simulink library "csu_tdl_thruster_dynamics_lander_lib"  (R2014b)
settings: Solver=ode45  StartTime=0.0  StopTime=10.0  RelTol=1e-3
values from neighbouring files (symbols this model uses):
  sim_time_step_size = 0.01    [csu_tdl_thruster_dynamics_lander_test.m]    (also in sim_thruster_wsim_test.m)
  tdl_active_time = 0.9/1000    (= 0.0009)    [csu_tdl_thruster_dynamics_lander_init.m]
undefined symbols (not defined in the file or in its folder): tdl_valve_delay_cycles
libraries: simulink x7, util_event_lib x2, util_info_lib x1, util_common_lib x1
settings Model: Creator=Nilesh  LastModifiedBy=mstewart

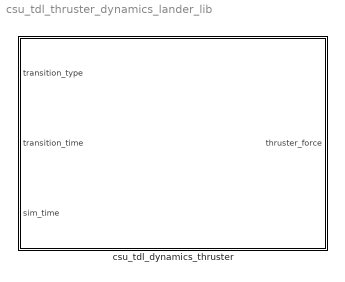
== system csu_tdl_thruster_dynamics_lander_lib ==
  csu_tdl_dynamics_thruster : Subsystem  mask{thruster_idx=[], num_thrusters=[], time_since_rise_lookup=[], thrust_rising_output_lookup=[], time_since_fall_lookup=[], thrust_falling_output_lookup=[], thrust_noise_mean=[], thrust_noise_std=[], thrust_noise_seed=[], thrust_noise_on=[]}
      mask prompts: thruster_idx "Thruster Index (1-total)"; num_thrusters "Number of thrusters (total)"; time_since_rise_lookup "Rising Transition: time vector for lookup table (seconds)"; thrust_rising_output_lookup "Rising Transition: thrust vector for lookup table (Newtons)"; time_since_fall_lookup "Falling Transition: time vector for lookup table (seconds)"; thrust_falling_output_lookup "Falling Transition: thrust vector for lookup table (Newtons)"; thrust_noise_mean "Output noise: bias in Newtons"; thrust_noise_std "Output noise: standard deviation in Newtons"; thrust_noise_seed "Output noise: random seed"; thrust_noise_on "Outpur noise Enabled (1 is noisy, 0 is clean)"

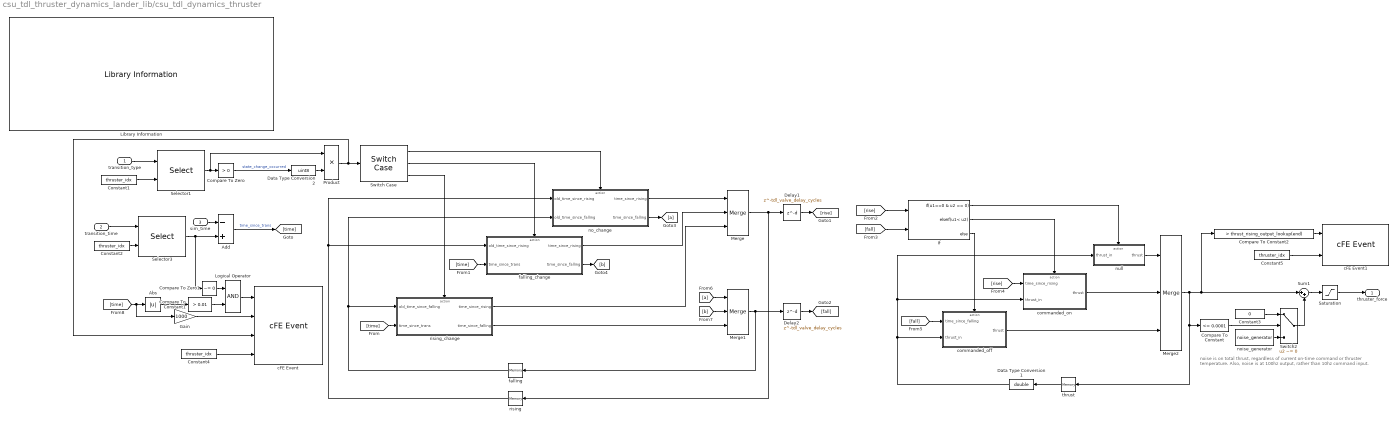
== system csu_tdl_thruster_dynamics_lander_lib/csu_tdl_dynamics_thruster ==
  note: noise is on total thrust, regardless of current on-time
      | command or thruster temperature. Also, noise is at 100hz output,
      | rather than 10hz command input.
  transition_type : Inport
  transition_time : Inport  Port=2
  sim_time : Inport  Port=3
  Abs : Abs
  Add : Sum  Inputs=-+
  Compare To Constant : simulink/Logic and Bit Operations/Compare To Constant  relop=<=  const=0.0001  OutDataTypeStr=boolean
  Compare To Constant1 : simulink/Logic and Bit Operations/Compare To Constant  relop=>  const=0.01  OutDataTypeStr=boolean
  Compare To Constant2 : simulink/Logic and Bit Operations/Compare To Constant  relop=>  const=thrust_rising_output_lookup(end)  OutDataTypeStr=boolean
  Compare To Zero : simulink/Logic and Bit Operations/Compare To Zero  relop=>  OutDataTypeStr=boolean
  Compare To Zero1 : simulink/Logic and Bit Operations/Compare To Zero  relop=~=  OutDataTypeStr=boolean
  Constant{1..2,4..5} (4 alike) : Constant  Value=thruster_idx  OutDataTypeStr=uint8
  Constant3 : Constant  Value=0
  Data Type Conversion1 : DataTypeConversion  OutDataTypeStr=double
  Data Type Conversion2 : DataTypeConversion  OutDataTypeStr=uint8
  Delay1 : Delay  DelayLength=tdl_valve_delay_cycles
  Delay2 : Delay  DelayLength=tdl_valve_delay_cycles
  Gain : Gain  Gain=1000
  If : If  NumInputs=2  IfExpression=u1==0 & u2 == 0  ElseIfExpressions=u1< u2
  Library Information : util_info_lib/Library Information  owner='escrane'
  Logical Operator : Logic  AllPortsSameDT=off  OutDataTypeStr=boolean
  Merge : Merge  Inputs=3
  Merge1 : Merge  Inputs=3
  Merge2 : Merge  Inputs=3
  Product : Product
  Saturation : Saturate  UpperLimit=1e10  LowerLimit=0
  Selector1 : Selector  InputPortWidth=num_thrusters  IndexOptions=Index vector (port)  Indices=[1 3]
  Selector3 : Selector  InputPortWidth=num_thrusters  IndexOptions=Index vector (port)  Indices=[1 3]
  Sum1 : Sum  Inputs=|++
  Switch Case : SwitchCase  CaseConditions={0,1,2}  ShowDefaultCase=off
  Switch2 : Switch  Criteria=u2 ~= 0
  cFE Event : util_event_lib/cFE Event  event_message='Incorrect transition time %f milliseconds detected on transition type %u in thruster %u'  event_id=thruster_idx+20  event_severity=DEBUG  event_use_enums=off  event_enum_types={}
  cFE Event1 : util_event_lib/cFE Event  event_message='Large thrust output in thruster %u'  event_id=thruster_idx+50  event_severity=DEBUG  event_use_enums=off  event_enum_types={}
  commanded_off : Subsystem  TreatAsAtomicUnit=on
  commanded_on : Subsystem  TreatAsAtomicUnit=on
  falling : Memory  InheritSampleTime=on
  falling_change : Subsystem  TreatAsAtomicUnit=on
  no_change : Subsystem  TreatAsAtomicUnit=on
  noise_generator : util_common_lib/noise_generator  std_dev=thrust_noise_std  bias=thrust_noise_mean  seed=thrust_noise_seed  on=thrust_noise_on  sample_time=sim_time_step_size
  null : Subsystem  TreatAsAtomicUnit=on
  rising : Memory  InheritSampleTime=on
  rising_change : Subsystem  TreatAsAtomicUnit=on
  thrust : Memory  InheritSampleTime=on
  thruster_force : Outport
  wires:
  If/1 -> null/Action
  thrust/1 -> Data Type Conversion1/1
  null/1(thrust) -> Merge2/1
  commanded_on/1(thrust) -> Merge2/2
  commanded_off/1(thrust) -> Merge2/3
  If/2 -> commanded_on/Action
  Delay2/1 -> [fall]
  Delay1/1 -> [rise]
  Merge1/1 -> falling/1, Delay2/1
  Merge/1 -> rising/1, Delay1/1
  [b] -> Merge1/2
  falling_change/2(time_since_falling) -> [b]
  [a] -> Merge1/1
  no_change/2(time_since_falling) -> [a]
  no_change/1(time_since_rising) -> Merge/1
  [fall] -> commanded_off/1(time_since_falling)
  [rise] -> commanded_on/1(time_since_rising)
  If/3 -> commanded_off/Action
  [rise] -> If/1
  [fall] -> If/2
  sim_time/1 -> Add/1
  Compare To Zero/1 -> Data Type Conversion2/1  "state_change_occurred"
  Data Type Conversion2/1 -> Product/2
  Add/1 -> [time]  "time_since_trans"
  Product/1 -> cFE Event/3, Switch Case/1
  Switch Case/1 -> no_change/Action
  Switch Case/2 -> falling_change/Action
  Switch Case/3 -> rising_change/Action
  [time] -> rising_change/2(time_since_trans)
  [time] -> falling_change/2(time_since_trans)
  falling/1 -> rising_change/1(old_time_since_falling), no_change/2(old_time_since_falling)
  rising/1 -> falling_change/1(old_time_since_rising), no_change/1(old_time_since_rising)
  falling_change/1(time_since_rising) -> Merge/2
  rising_change/1(time_since_rising) -> Merge/3
  rising_change/2(time_since_falling) -> Merge1/3
  Constant2/1 -> Selector3/2
  transition_time/1 -> Selector3/1
  Selector3/1 -> Compare To Zero1/1, Add/2
  Constant1/1 -> Selector1/2
  transition_type/1 -> Selector1/1
  Selector1/1 -> Product/1, Compare To Zero/1
  Data Type Conversion1/1 -> commanded_off/2(thrust_in), commanded_on/2(thrust_in), null/1(thrust_in)
  Compare To Constant/1 -> Switch2/2
  noise_generator/1 -> Switch2/3
  Constant3/1 -> Switch2/1
  Sum1/1 -> Saturation/1
  Switch2/1 -> Sum1/2
  Saturation/1 -> thruster_force/1
  [time] -> Abs/1, Gain/1
  Abs/1 -> Compare To Constant1/1
  Compare To Zero1/1 -> Logical Operator/1
  Compare To Constant1/1 -> Logical Operator/2
  Logical Operator/1 -> cFE Event/1
  Constant4/1 -> cFE Event/4
  Merge2/1 -> Compare To Constant2/1, Sum1/1, thrust/1, Compare To Constant/1
  Compare To Constant2/1 -> cFE Event1/1
  Constant5/1 -> cFE Event1/2
  Gain/1 -> cFE Event/2

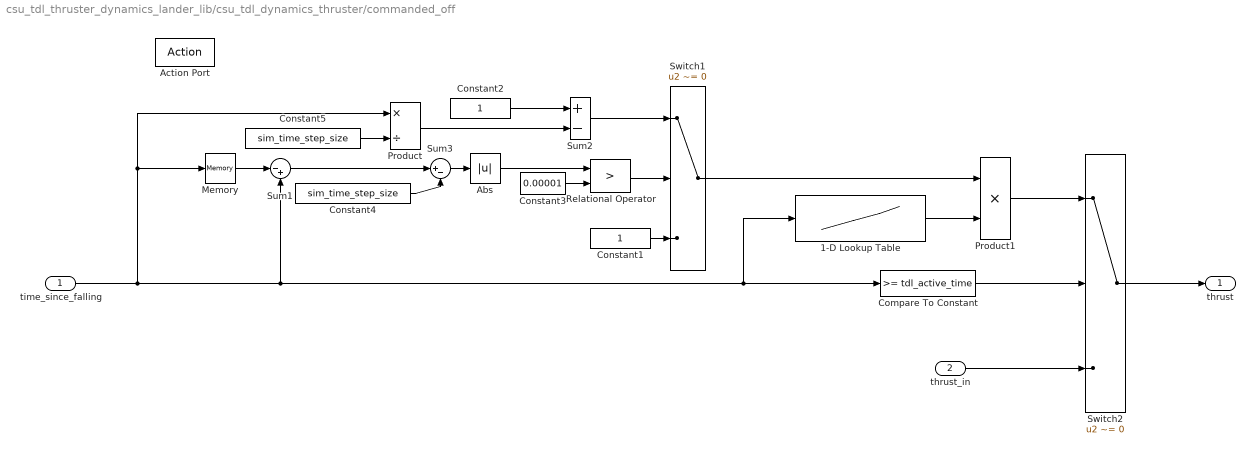
== system csu_tdl_thruster_dynamics_lander_lib/csu_tdl_dynamics_thruster/commanded_off ==
  time_since_falling : Inport
  thrust_in : Inport  Port=2
  Action Port : ActionPort
  1-D Lookup Table : Lookup_n-D  NumberOfTableDimensions=1  BreakpointsForDimension1=time_since_fall_lookup  BeginIndexSearchUsingPreviousIndexResult=on  Table=thrust_falling_output_lookup  ExtrapMethod=Clip  UseLastTableValue=on  InternalRulePriority=Speed  RndMeth=Simplest  InputSameDT=on
  Abs : Abs
  Compare To Constant : simulink/Logic and Bit Operations/Compare To Constant  relop=>=  const=tdl_active_time  OutDataTypeStr=boolean
  Constant1 : Constant
  Constant2 : Constant
  Constant3 : Constant  Value=0.00001  OutDataTypeStr=double
  Constant4 : Constant  Value=sim_time_step_size
  Constant5 : Constant  Value=sim_time_step_size
  Memory : Memory  InheritSampleTime=on
  Product : Product  Inputs=*/
  Product1 : Product
  Relational Operator : RelationalOperator  Operator=>  OutDataTypeStr=boolean
  Sum1 : Sum  Inputs=|-+
  Sum2 : Sum  Inputs=+-
  Sum3 : Sum  Inputs=|+-
  Switch1 : Switch  Criteria=u2 ~= 0
  Switch2 : Switch  Criteria=u2 ~= 0
  thrust : Outport  InitialOutput=0
  wires:
  Switch2/1 -> thrust/1
  thrust_in/1 -> Switch2/3
  Compare To Constant/1 -> Switch2/2
  time_since_falling/1 -> Memory/1, Product/1, Sum1/2, Compare To Constant/1, 1-D Lookup Table/1
  Constant5/1 -> Product/2
  Memory/1 -> Sum1/1
  Relational Operator/1 -> Switch1/2
  Constant1/1 -> Switch1/3
  Sum2/1 -> Switch1/1
  Product/1 -> Sum2/2
  Constant2/1 -> Sum2/1
  Sum1/1 -> Sum3/1
  Constant4/1 -> Sum3/2
  Sum3/1 -> Abs/1
  Abs/1 -> Relational Operator/1
  Constant3/1 -> Relational Operator/2
  Switch1/1 -> Product1/1
  1-D Lookup Table/1 -> Product1/2
  Product1/1 -> Switch2/1

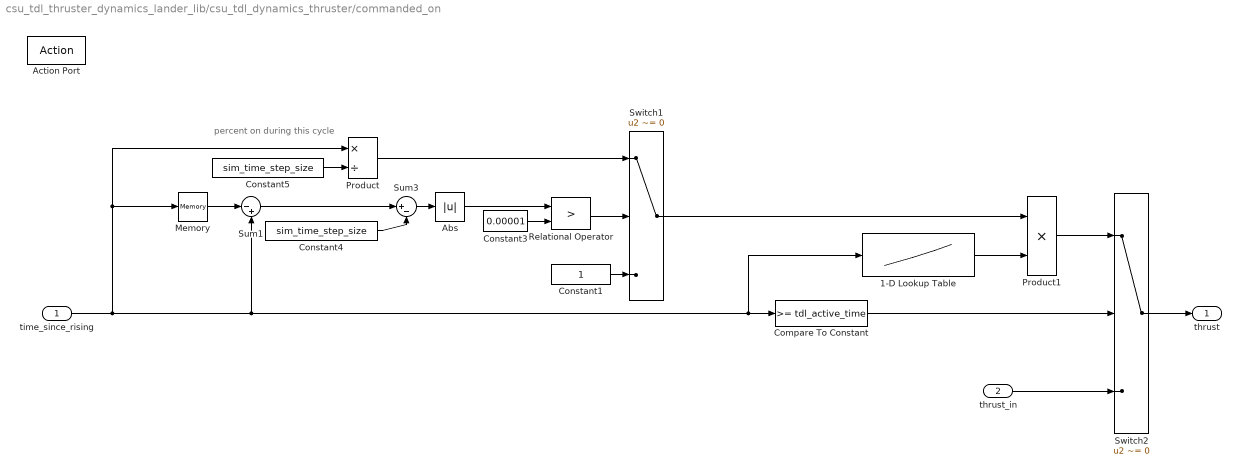
== system csu_tdl_thruster_dynamics_lander_lib/csu_tdl_dynamics_thruster/commanded_on ==
  note: percent on during this cycle
  time_since_rising : Inport
  thrust_in : Inport  Port=2
  Action Port : ActionPort
  1-D Lookup Table : Lookup_n-D  NumberOfTableDimensions=1  BreakpointsForDimension1=time_since_rise_lookup  BeginIndexSearchUsingPreviousIndexResult=on  Table=thrust_rising_output_lookup  ExtrapMethod=Clip  UseLastTableValue=on  InternalRulePriority=Speed  RndMeth=Simplest  InputSameDT=on
  Abs : Abs
  Compare To Constant : simulink/Logic and Bit Operations/Compare To Constant  relop=>=  const=tdl_active_time  OutDataTypeStr=boolean
  Constant1 : Constant
  Constant3 : Constant  Value=0.00001  OutDataTypeStr=double
  Constant4 : Constant  Value=sim_time_step_size
  Constant5 : Constant  Value=sim_time_step_size
  Memory : Memory  InheritSampleTime=on
  Product : Product  Inputs=*/
  Product1 : Product
  Relational Operator : RelationalOperator  Operator=>  OutDataTypeStr=boolean
  Sum1 : Sum  Inputs=|-+
  Sum3 : Sum  Inputs=|+-
  Switch1 : Switch  Criteria=u2 ~= 0
  Switch2 : Switch  Criteria=u2 ~= 0
  thrust : Outport  InitialOutput=0
  wires:
  Switch2/1 -> thrust/1
  thrust_in/1 -> Switch2/3
  Compare To Constant/1 -> Switch2/2
  time_since_rising/1 -> Product/1, Memory/1, 1-D Lookup Table/1, Compare To Constant/1, Sum1/2
  1-D Lookup Table/1 -> Product1/2
  Product1/1 -> Switch2/1
  Constant5/1 -> Product/2
  Memory/1 -> Sum1/1
  Constant1/1 -> Switch1/3
  Switch1/1 -> Product1/1
  Sum1/1 -> Sum3/1
  Constant4/1 -> Sum3/2
  Sum3/1 -> Abs/1
  Abs/1 -> Relational Operator/1
  Constant3/1 -> Relational Operator/2
  Relational Operator/1 -> Switch1/2
  Product/1 -> Switch1/1

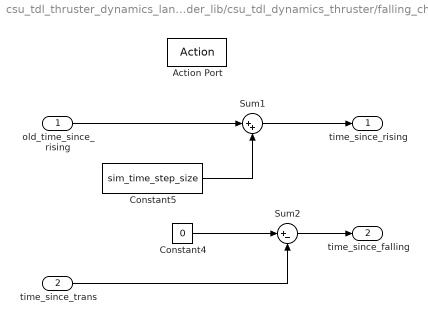
== system csu_tdl_thruster_dynamics_lander_lib/csu_tdl_dynamics_thruster/falling_change ==
  old_time_since_rising : Inport
  time_since_trans : Inport  Port=2
  Action Port : ActionPort
  Constant4 : Constant  Value=0
  Constant5 : Constant  Value=sim_time_step_size
  Sum1 : Sum  Inputs=|++
  Sum2 : Sum  Inputs=|+-
  time_since_rising : Outport
  time_since_falling : Outport  Port=2
  wires:
  Constant4/1 -> Sum2/1
  Sum1/1 -> time_since_rising/1
  old_time_since_rising/1 -> Sum1/1
  Constant5/1 -> Sum1/2
  time_since_trans/1 -> Sum2/2
  Sum2/1 -> time_since_falling/1

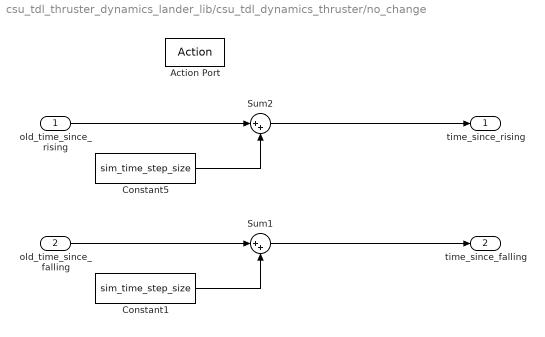
== system csu_tdl_thruster_dynamics_lander_lib/csu_tdl_dynamics_thruster/no_change ==
  old_time_since_rising : Inport
  old_time_since_falling : Inport  Port=2
  Action Port : ActionPort
  Constant1 : Constant  Value=sim_time_step_size
  Constant5 : Constant  Value=sim_time_step_size
  Sum1 : Sum  Inputs=|++
  Sum2 : Sum  Inputs=|++
  time_since_rising : Outport
  time_since_falling : Outport  Port=2
  wires:
  old_time_since_rising/1 -> Sum2/1
  Constant5/1 -> Sum2/2
  Sum2/1 -> time_since_rising/1
  old_time_since_falling/1 -> Sum1/1
  Constant1/1 -> Sum1/2
  Sum1/1 -> time_since_falling/1

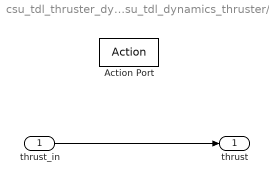
== system csu_tdl_thruster_dynamics_lander_lib/csu_tdl_dynamics_thruster/null ==
  thrust_in : Inport
  Action Port : ActionPort
  thrust : Outport  InitialOutput=0
  wires:
  thrust_in/1 -> thrust/1

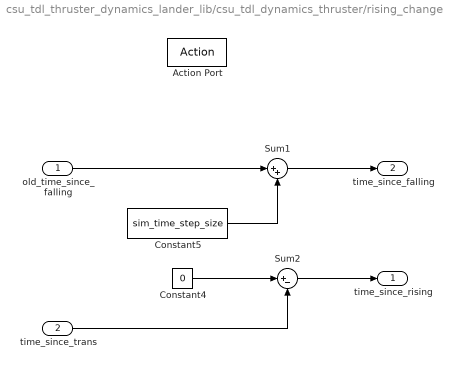
== system csu_tdl_thruster_dynamics_lander_lib/csu_tdl_dynamics_thruster/rising_change ==
  old_time_since_falling : Inport
  time_since_trans : Inport  Port=2
  Action Port : ActionPort
  Constant4 : Constant  Value=0
  Constant5 : Constant  Value=sim_time_step_size
  Sum1 : Sum  Inputs=|++
  Sum2 : Sum  Inputs=|+-
  time_since_rising : Outport
  time_since_falling : Outport  Port=2
  wires:
  Sum2/1 -> time_since_rising/1
  Constant4/1 -> Sum2/1
  time_since_trans/1 -> Sum2/2
  old_time_since_falling/1 -> Sum1/1
  Sum1/1 -> time_since_falling/1
  Constant5/1 -> Sum1/2
